simulink model "Test"  (R2021a)
settings: Solver=VariableStepAuto  StartTime=0.0  StopTime=10.0  RelTol=1e-3
values from neighbouring files (symbols this model uses):
  ff = 1.1    [Linearize_Fast.m]
  g = 9.81    [Linearize_Fast.m]    (also in Param_set.m = 9.8)
  ground_alt = 180.2070    (= 180.207)    [Linearize_Fast.m]
  m = 0.068    [Param_set.m]
  Mixer = double(subs(n_lin, [u_vec; a; b; c; d;], [.66708; 0; 0; 0;(1.86e-6);(8.856e-8);(8.856e-8);(9.766e-9)]))    [Linearize_Fast.m]
undefined symbols (not defined in the file or in its folder): all_cov, Discrete, K_PD, K_psi, K_u, K_v, Time
libraries: simulink x9, ctrlSharedLib x5
settings Model: Creator=jtc12  LastModifiedBy=jtc12

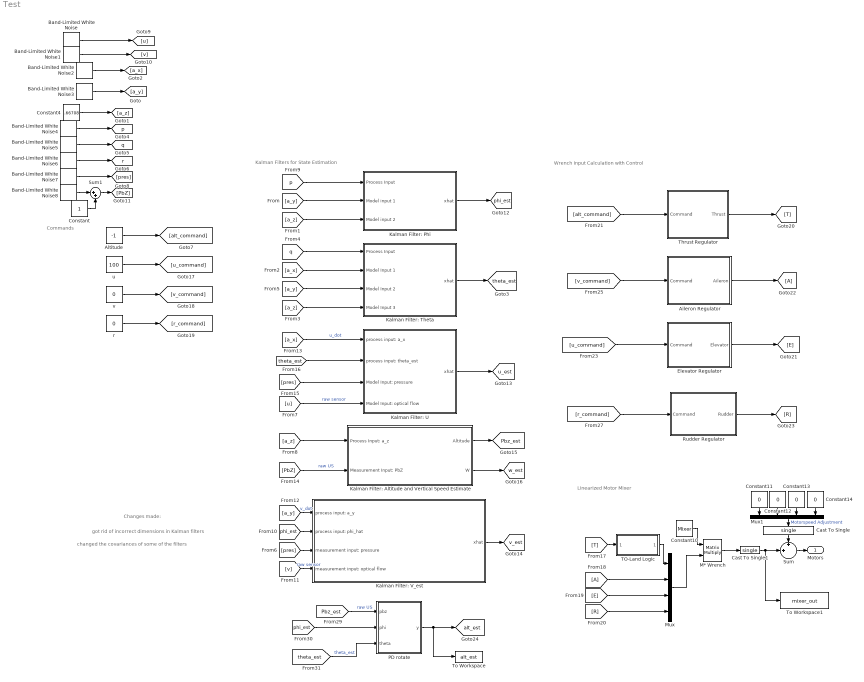
== system Test ==
  note: changed the covariances of some of the filters
  note: got rid of incorrect dimensions in Kalman filters
  note: Changes made:
  note: Commands
  note: Kalman Filters for State Estimation
  note: Wrench Input Calculation with Control
  note: Linearized Motor Mixer
  Aileron Regulator : Subsystem
  Altitude : Constant  Value=-1
  Band-Limited White Noise{,1..8} (9 alike) : simulink/Sources/Band-Limited White Noise  Cov=[0.1]  Ts=1/200  seed=[23341]
  Cast To Single : DataTypeConversion  OutDataTypeStr=single
  Cast To Single1 : DataTypeConversion  OutDataTypeStr=single
  Constant : Constant
  Constant10 : Constant  Value=Mixer
  Constant{11..14} (4 alike) : Constant  Value=0
  Constant4 : Constant  Value=.66708
  Elevator Regulator : Subsystem
  Kalman Filter: Altitude and Vertical Speed Estimate : Subsystem
  Kalman Filter: Phi : Subsystem
  Kalman Filter: Theta : Subsystem
  Kalman Filter: U : Subsystem
  Kalman Filter: V_est : Subsystem
  M* Wrench : Product  Multiplication=Matrix(*)
  Mux : Mux
  Mux1 : Mux
  PD rotate : MATLAB Function  TreatAsAtomicUnit=on
  Rudder Regulator : Subsystem
  Sum : Sum  Inputs=+|+||
  Sum1 : Sum  Inputs=|++
  TO-Land Logic : Subsystem
  Thrust Regulator : Subsystem
  To Workspace : ToWorkspace  VariableName=alt_est  SaveFormat=Timeseries  SampleTime=-1
  To Workspace1 : ToWorkspace  VariableName=mixer_out  SaveFormat=Timeseries  SampleTime=-1
  r : Constant  Value=0
  u : Constant  Value=100
  v : Constant  Value=0
  Motors : Outport  VectorParamsAs1DForOutWhenUnconnected=off
  tag scope: Pbz_est=global, alt_est=global, p=global, phi_est=global, q=global, r=global, theta_est=global, u_est=global, v_est=global, w_est=global
  wires:
  Band-Limited White Noise2/1 -> [a_x]
  Band-Limited White Noise3/1 -> [a_y]
  Constant4/1 -> [a_z]
  Band-Limited White Noise5/1 -> [q]
  Band-Limited White Noise6/1 -> [r]
  Band-Limited White Noise7/1 -> [pres]
  Altitude/1 -> [alt_command]
  v/1 -> [v_command]
  u/1 -> [u_command]
  r/1 -> [r_command]
  [phi_est] -> PD rotate/2(phi)
  [a_x] -> Kalman Filter: Theta/2(Model Input 1)
  Kalman Filter: Altitude and Vertical Speed Estimate/1(Altitude) -> [Pbz_est]
  Kalman Filter: V_est/1(xhat) -> [v_est]
  [PbZ] -> Kalman Filter: Altitude and Vertical Speed Estimate/2(Measurement Input: PbZ)  "raw US"
  [theta_est] -> PD rotate/3(theta)  "theta_est"
  Kalman Filter: Altitude and Vertical Speed Estimate/2(W) -> [w_est]
  [pres] -> Kalman Filter: V_est/3(measurement input: pressure)
  [Pbz_est] -> PD rotate/1(pbz)  "raw US"
  [a_y] -> Kalman Filter: Theta/3(Model Input 2)
  [a_z] -> Kalman Filter: Theta/4(Model Input 3)
  [a_y] -> Kalman Filter: Phi/2(Model input 1)
  [u] -> Kalman Filter: U/4(Model Input: optical flow)  "raw sensor"
  [pres] -> Kalman Filter: U/3(Model Input: pressure)
  [q] -> Kalman Filter: Theta/1(Process Input)
  Kalman Filter: U/1(xhat) -> [u_est]
  [a_y] -> Kalman Filter: V_est/1("process input: a_y   ")  "v_dot"
  [phi_est] -> Kalman Filter: V_est/2("process input: phi_hat ")
  [a_z] -> Kalman Filter: Altitude and Vertical Speed Estimate/1("Process Input: a_z ")
  Kalman Filter: Theta/1(xhat) -> [theta_est]
  [a_x] -> Kalman Filter: U/1(process input: a_x)  "u_dot"
  Kalman Filter: Phi/1(xhat) -> [phi_est]
  [theta_est] -> Kalman Filter: U/2(process input: theta_est)
  [a_z] -> Kalman Filter: Phi/3(Model input 2)
  PD rotate/1(y) -> To Workspace/1, [alt_est]
  [p] -> Kalman Filter: Phi/1(Process Input)
  [v] -> Kalman Filter: V_est/4(measurement input: optical flow)  "raw sensor"
  Rudder Regulator/1(Rudder) -> [R]
  Aileron Regulator/1(Aileron) -> [A]
  Thrust Regulator/1(Thrust) -> [T]
  [u_command] -> Elevator Regulator/1(Command)
  [alt_command] -> Thrust Regulator/1(Command)
  Elevator Regulator/1(Elevator) -> [E]
  [v_command] -> Aileron Regulator/1(Command)
  [r_command] -> Rudder Regulator/1(Command)
  Constant13/1 -> Mux1/3
  Constant12/1 -> Mux1/2
  Mux/1 -> M* Wrench/2
  [R] -> Mux/4
  Cast To Single1/1 -> Sum/2, To Workspace1/1
  Mux1/1 -> Cast To Single/1  "Motorspeed Adjustment"
  [E] -> Mux/3
  Cast To Single/1 -> Sum/1
  [T] -> TO-Land Logic/1(Thrust In)
  M* Wrench/1 -> Cast To Single1/1
  [A] -> Mux/2
  Constant10/1 -> M* Wrench/1
  Constant14/1 -> Mux1/4
  Sum/1 -> Motors/1
  TO-Land Logic/1(Thrust Out) -> Mux/1
  Constant11/1 -> Mux1/1
  Band-Limited White Noise/1 -> [u]
  Band-Limited White Noise1/1 -> [v]
  Band-Limited White Noise4/1 -> [p]
  Band-Limited White Noise8/1 -> Sum1/1
  Sum1/1 -> [PbZ]
  Constant/1 -> Sum1/2

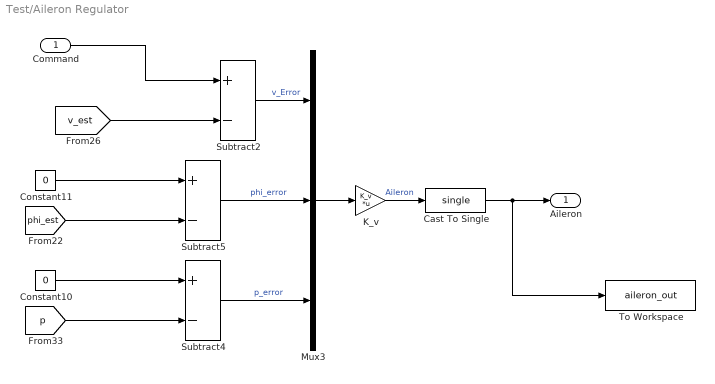
== system Test/Aileron Regulator ==
  Command : Inport
  Cast To Single : DataTypeConversion  OutDataTypeStr=single
  Constant10 : Constant  Value=0
  Constant11 : Constant  Value=0
  K_v : Gain  Gain=K_v  Multiplication=Matrix(K*u)
  Mux3 : Mux  Inputs=3
  Subtract2 : Sum  Inputs=+-
  Subtract4 : Sum  Inputs=+-
  Subtract5 : Sum  Inputs=+-
  To Workspace : ToWorkspace  VariableName=aileron_out  SaveFormat=Timeseries  SampleTime=-1
  Aileron : Outport
  wires:
  [p] -> Subtract4/2
  [v_est] -> Subtract2/2
  Constant11/1 -> Subtract5/1
  [phi_est] -> Subtract5/2
  Subtract5/1 -> Mux3/2  "phi_error"
  Subtract2/1 -> Mux3/1  "v_Error"
  Mux3/1 -> K_v/1
  Subtract4/1 -> Mux3/3  "p_error"
  Constant10/1 -> Subtract4/1
  K_v/1 -> Cast To Single/1  "Aileron"
  Command/1 -> Subtract2/1
  Cast To Single/1 -> To Workspace/1, Aileron/1

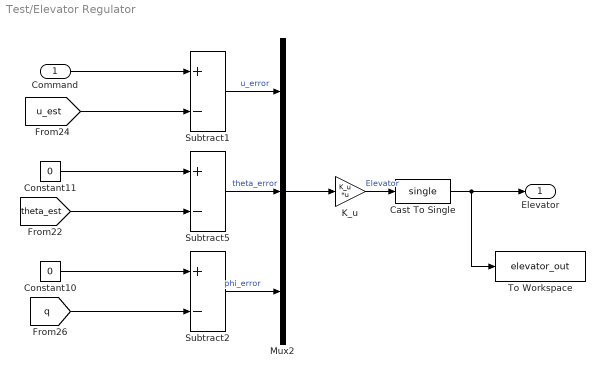
== system Test/Elevator Regulator ==
  Command : Inport
  Cast To Single : DataTypeConversion  OutDataTypeStr=single
  Constant10 : Constant  Value=0
  Constant11 : Constant  Value=0
  K_u : Gain  Gain=K_u  Multiplication=Matrix(K*u)
  Mux2 : Mux  Inputs=3
  Subtract1 : Sum  Inputs=+-
  Subtract2 : Sum  Inputs=+-
  Subtract5 : Sum  Inputs=+-
  To Workspace : ToWorkspace  VariableName=elevator_out  SaveFormat=Timeseries  SampleTime=-1
  Elevator : Outport
  wires:
  [theta_est] -> Subtract5/2
  [u_est] -> Subtract1/2
  Constant10/1 -> Subtract2/1
  Constant11/1 -> Subtract5/1
  Subtract5/1 -> Mux2/2  "theta_error"
  Subtract1/1 -> Mux2/1  "u_error"
  Subtract2/1 -> Mux2/3  "phi_error"
  Mux2/1 -> K_u/1
  [q] -> Subtract2/2
  K_u/1 -> Cast To Single/1  "Elevator"
  Command/1 -> Subtract1/1
  Cast To Single/1 -> To Workspace/1, Elevator/1

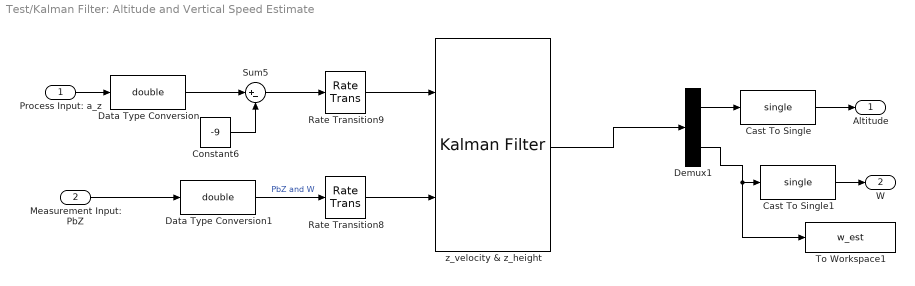
== system Test/Kalman Filter: Altitude and Vertical Speed Estimate ==
  "Process Input: a_z " : Inport
  Measurement Input: PbZ : Inport  Port=2
  Cast To Single : DataTypeConversion  OutDataTypeStr=single
  Cast To Single1 : DataTypeConversion  OutDataTypeStr=single
  Constant6 : Constant  Value=-9
  Data Type Conversion : DataTypeConversion  OutDataTypeStr=double
  Data Type Conversion1 : DataTypeConversion  OutDataTypeStr=double
  Demux1 : Demux  Outputs=2
  Rate Transition8 : RateTransition  OutPortSampleTime=1/200
  Rate Transition9 : RateTransition  OutPortSampleTime=1/200
  Sum5 : Sum  Inputs=|+-
  To Workspace1 : ToWorkspace  VariableName=w_est  SaveFormat=Timeseries  SampleTime=-1
  z_velocity & z_height : ctrlSharedLib/Kalman Filter  TimeDomain=Discrete-Time  UseCurrentEstimator=on  ModelSource=Individual A, B, C, D matrices  ModelSourceVariable=ss(0.95,1,1,0,1)  A=[1 1/200;0 1]  B=[0; 1/200]  C=[1 0]  D=0  NumberOfStates=1  NumberOfInputs=1  NumberOfOutputs=1  InitialEstimateSource=Dialog  X0=0  P0=10  UseK=off  UseGH=off  NumberOfProcessNoiseInputs=1  G=1  TimeInvariantG=on  H=0  TimeInvariantH=on  Q=all_cov(7,7)/1000  TimeInvariantQ=on  R=all_cov(1,1)  TimeInvariantR=on  N=0  TimeInvariantN=on  AddInputPort=on  AddEnablePort=off  OutputEstimatedY=off  OutputP=off  Ts=-1
  Altitude : Outport
  W : Outport  Port=2
  wires:
  Data Type Conversion1/1 -> Rate Transition8/1  "PbZ and W"
  Constant6/1 -> Sum5/2
  Demux1/1 -> Cast To Single/1
  Sum5/1 -> Rate Transition9/1
  Data Type Conversion/1 -> Sum5/1
  Rate Transition9/1 -> z_velocity & z_height/1
  Rate Transition8/1 -> z_velocity & z_height/2
  Measurement Input: PbZ/1 -> Data Type Conversion1/1
  Demux1/2 -> Cast To Single1/1, To Workspace1/1
  "Process Input: a_z "/1 -> Data Type Conversion/1
  z_velocity & z_height/1 -> Demux1/1
  Cast To Single/1 -> Altitude/1
  Cast To Single1/1 -> W/1

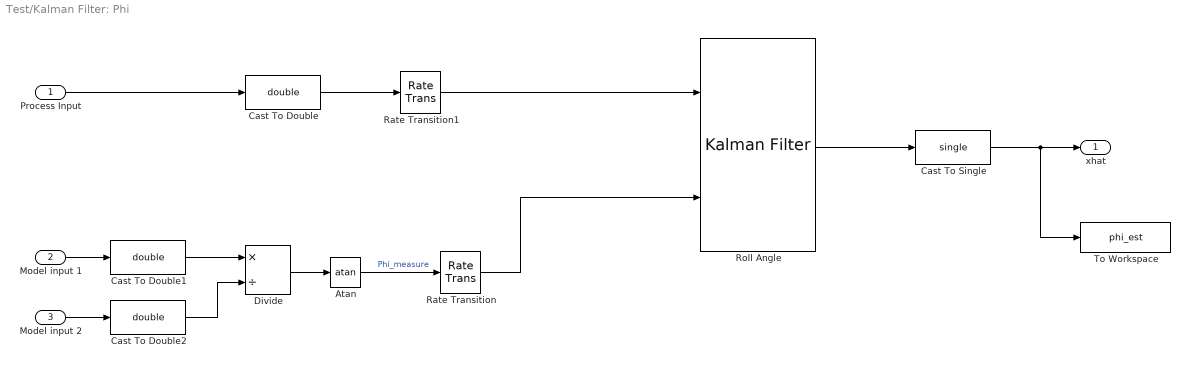
== system Test/Kalman Filter: Phi ==
  Process Input : Inport
  Model input 1 : Inport  Port=2
  Model input 2 : Inport  Port=3
  Atan : Trigonometry  Operator=atan
  Cast To Double : DataTypeConversion  OutDataTypeStr=double
  Cast To Double1 : DataTypeConversion  OutDataTypeStr=double
  Cast To Double2 : DataTypeConversion  OutDataTypeStr=double
  Cast To Single : DataTypeConversion  OutDataTypeStr=single
  Divide : Product  Inputs=*/
  Rate Transition : RateTransition  OutPortSampleTime=1/200
  Rate Transition1 : RateTransition  OutPortSampleTime=1/200
  Roll Angle : ctrlSharedLib/Kalman Filter  TimeDomain=Discrete-Time  UseCurrentEstimator=on  ModelSource=Individual A, B, C, D matrices  ModelSourceVariable=ss(0.95,1,1,0,1)  A=[1]  B=[1/200]  C=[1]  D=0  NumberOfStates=1  NumberOfInputs=1  NumberOfOutputs=1  InitialEstimateSource=Dialog  X0=0  P0=10  UseK=off  UseGH=off  NumberOfProcessNoiseInputs=1  G=1  TimeInvariantG=on  H=0  TimeInvariantH=on  Q=.0133/200  TimeInvariantQ=on  R=.0101  TimeInvariantR=on  N=0  TimeInvariantN=on  AddInputPort=on  AddEnablePort=off  OutputEstimatedY=off  OutputP=off  Ts=-1
  To Workspace : ToWorkspace  VariableName=phi_est  SaveFormat=Timeseries  SampleTime=-1
  xhat : Outport
  wires:
  Divide/1 -> Atan/1
  Atan/1 -> Rate Transition/1  "Phi_measure"
  Process Input/1 -> Cast To Double/1
  Rate Transition/1 -> Roll Angle/2
  Rate Transition1/1 -> Roll Angle/1
  Cast To Double/1 -> Rate Transition1/1
  Cast To Double1/1 -> Divide/1
  Model input 1/1 -> Cast To Double1/1
  Model input 2/1 -> Cast To Double2/1
  Cast To Double2/1 -> Divide/2
  Cast To Single/1 -> To Workspace/1, xhat/1
  Roll Angle/1 -> Cast To Single/1

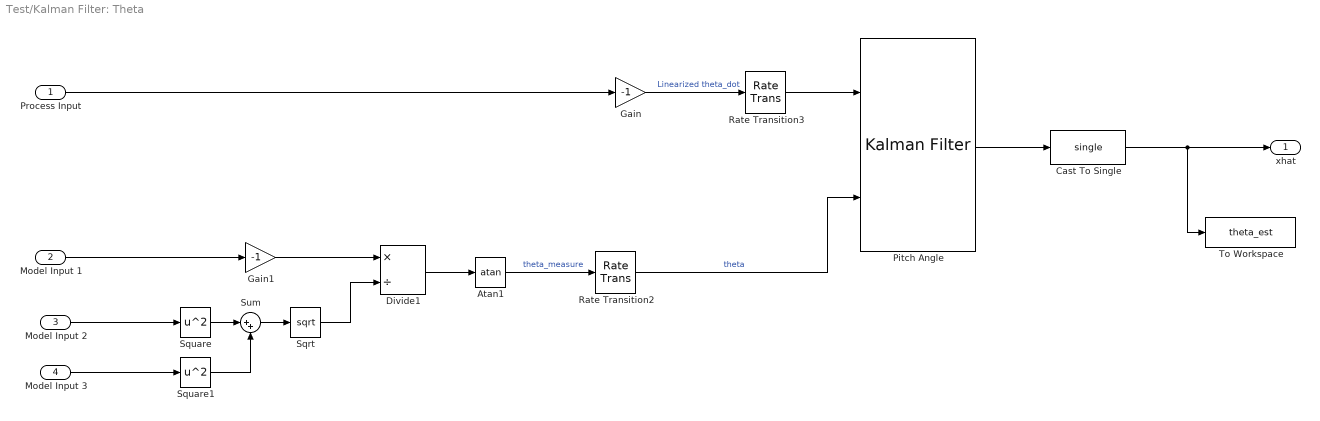
== system Test/Kalman Filter: Theta ==
  Process Input : Inport
  Model Input 1 : Inport  Port=2
  Model Input 2 : Inport  Port=3
  Model Input 3 : Inport  Port=4
  Atan1 : Trigonometry  Operator=atan
  Cast To Single : DataTypeConversion  OutDataTypeStr=single
  Divide1 : Product  Inputs=*/
  Gain : Gain  Gain=-1
  Gain1 : Gain  Gain=-1
  Pitch Angle : ctrlSharedLib/Kalman Filter  TimeDomain=Discrete-Time  UseCurrentEstimator=on  ModelSource=Individual A, B, C, D matrices  ModelSourceVariable=ss(0.95,1,1,0,1)  A=[1]  B=[1/200]  C=[1]  D=0  NumberOfStates=1  NumberOfInputs=1  NumberOfOutputs=1  InitialEstimateSource=Dialog  X0=0  P0=10  UseK=off  UseGH=off  NumberOfProcessNoiseInputs=1  G=1  TimeInvariantG=on  H=0  TimeInvariantH=on  Q=.0085/1000  TimeInvariantQ=on  R=.0066/10  TimeInvariantR=on  N=0  TimeInvariantN=on  AddInputPort=on  AddEnablePort=off  OutputEstimatedY=off  OutputP=off  Ts=-1
  Rate Transition2 : RateTransition  OutPortSampleTime=1/200
  Rate Transition3 : RateTransition  OutPortSampleTime=1/200
  Sqrt : Sqrt  SaturateOnIntegerOverflow=on
  Square : Math  Operator=square  SaturateOnIntegerOverflow=on
  Square1 : Math  Operator=square  SaturateOnIntegerOverflow=on
  Sum : Sum  Inputs=|++
  To Workspace : ToWorkspace  VariableName=theta_est  SaveFormat=Timeseries  SampleTime=-1
  xhat : Outport
  wires:
  Gain1/1 -> Divide1/1
  Divide1/1 -> Atan1/1
  Model Input 2/1 -> Square/1
  Rate Transition3/1 -> Pitch Angle/1
  Sum/1 -> Sqrt/1
  Square/1 -> Sum/1
  Square1/1 -> Sum/2
  Atan1/1 -> Rate Transition2/1  "theta_measure"
  Sqrt/1 -> Divide1/2
  Rate Transition2/1 -> Pitch Angle/2  "theta"
  Gain/1 -> Rate Transition3/1  "Linearized theta_dot"
  Process Input/1 -> Gain/1
  Model Input 1/1 -> Gain1/1
  Model Input 3/1 -> Square1/1
  Cast To Single/1 -> xhat/1, To Workspace/1
  Pitch Angle/1 -> Cast To Single/1

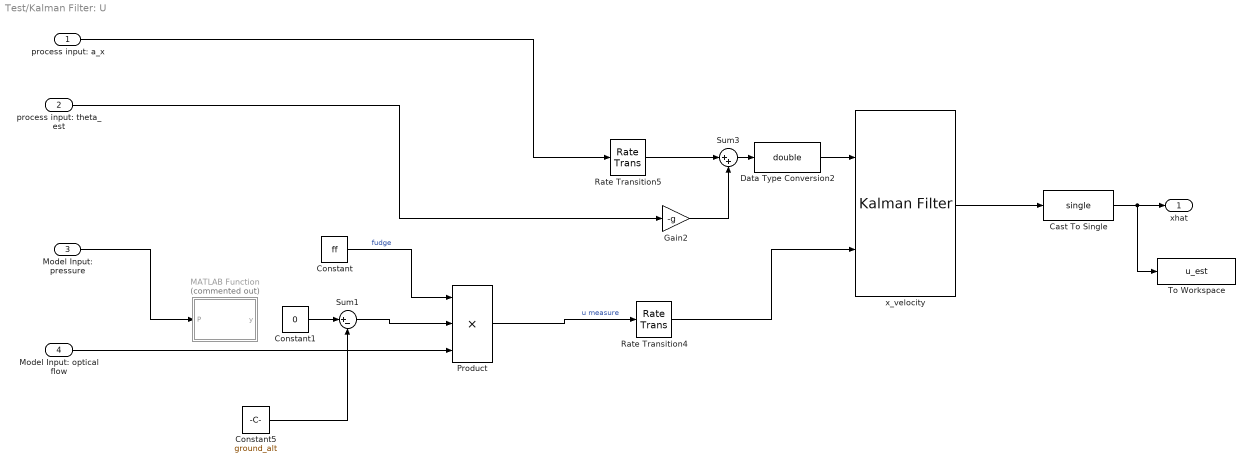
== system Test/Kalman Filter: U ==
  process input: a_x : Inport
  process input: theta_est : Inport  Port=2
  Model Input: pressure : Inport  Port=3
  Model Input: optical flow : Inport  Port=4
  Cast To Single : DataTypeConversion  OutDataTypeStr=single
  Constant : Constant  Value=ff
  Constant1 : Constant  Value=0
  Constant5 : Constant  Value=ground_alt
  Data Type Conversion2 : DataTypeConversion  OutDataTypeStr=double
  Gain2 : Gain  Gain=-g
  MATLAB Function : MATLAB Function  Commented=on  TreatAsAtomicUnit=on
  Product : Product  Inputs=3
  Rate Transition4 : RateTransition  OutPortSampleTime=1/200
  Rate Transition5 : RateTransition  OutPortSampleTime=1/200
  Sum1 : Sum  Inputs=|+-
  Sum3 : Sum  Inputs=|++
  To Workspace : ToWorkspace  VariableName=u_est  SaveFormat=Timeseries  SampleTime=-1
  x_velocity : ctrlSharedLib/Kalman Filter  TimeDomain=Discrete-Time  UseCurrentEstimator=on  ModelSource=Individual A, B, C, D matrices  ModelSourceVariable=ss(0.95,1,1,0,1)  A=[1]  B=[1/200]  C=[1]  D=0  NumberOfStates=1  NumberOfInputs=1  NumberOfOutputs=1  InitialEstimateSource=Dialog  X0=0  P0=10  UseK=off  UseGH=off  NumberOfProcessNoiseInputs=1  G=1  TimeInvariantG=on  H=0  TimeInvariantH=on  Q=.0059/200  TimeInvariantQ=on  R=all_cov(10,8)  TimeInvariantR=on  N=0  TimeInvariantN=on  AddInputPort=on  AddEnablePort=off  OutputEstimatedY=off  OutputP=off  Ts=-1
  xhat : Outport
  wires:
  process input: theta_est/1 -> Gain2/1
  Gain2/1 -> Sum3/2
  Product/1 -> Rate Transition4/1  "u measure"
  Rate Transition4/1 -> x_velocity/2
  process input: a_x/1 -> Rate Transition5/1
  Rate Transition5/1 -> Sum3/1
  Sum1/1 -> Product/2
  Data Type Conversion2/1 -> x_velocity/1
  Constant/1 -> Product/1  "fudge"
  Sum3/1 -> Data Type Conversion2/1
  Constant5/1 -> Sum1/2
  Model Input: pressure/1 -> MATLAB Function/1(P)
  Model Input: optical flow/1 -> Product/3
  Cast To Single/1 -> To Workspace/1, xhat/1
  x_velocity/1 -> Cast To Single/1
  Constant1/1 -> Sum1/1

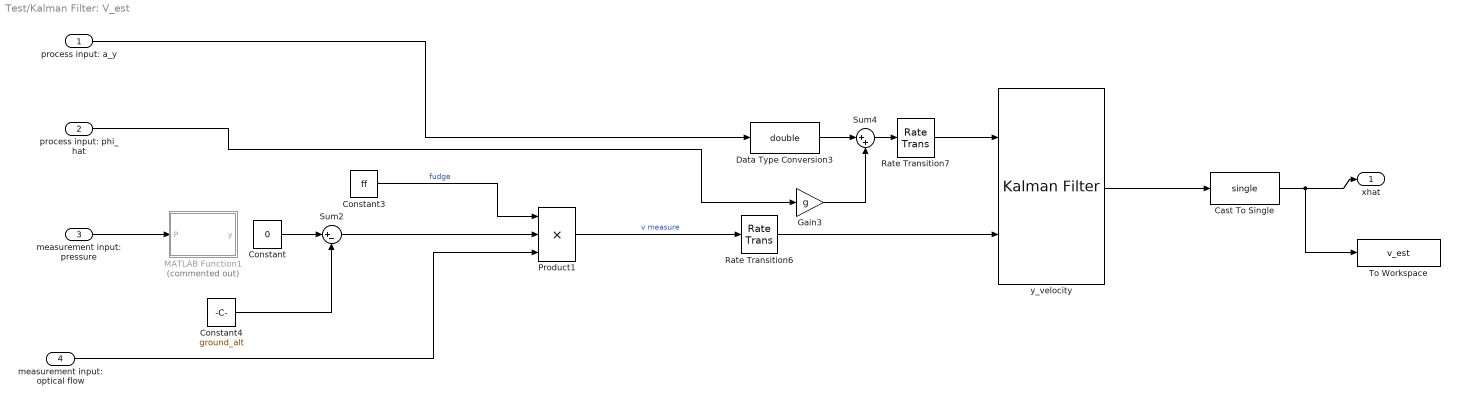
== system Test/Kalman Filter: V_est ==
  "process input: a_y   " : Inport
  "process input: phi_hat " : Inport  Port=2
  measurement input: pressure : Inport  Port=3
  measurement input: optical flow : Inport  Port=4
  Cast To Single : DataTypeConversion  OutDataTypeStr=single
  Constant : Constant  Value=0
  Constant3 : Constant  Value=ff
  Constant4 : Constant  Value=ground_alt
  Data Type Conversion3 : DataTypeConversion  OutDataTypeStr=double
  Gain3 : Gain  Gain=g
  MATLAB Function1 : MATLAB Function  Commented=on  TreatAsAtomicUnit=on
  Product1 : Product  Inputs=3
  Rate Transition6 : RateTransition  OutPortSampleTime=1/200
  Rate Transition7 : RateTransition  OutPortSampleTime=1/200
  Sum2 : Sum  Inputs=|+-
  Sum4 : Sum  Inputs=|++
  To Workspace : ToWorkspace  VariableName=v_est  SaveFormat=Timeseries  SampleTime=-1
  y_velocity : ctrlSharedLib/Kalman Filter  TimeDomain=Discrete-Time  UseCurrentEstimator=on  ModelSource=Individual A, B, C, D matrices  ModelSourceVariable=ss(0.95,1,1,0,1)  A=[1]  B=[1/200]  C=[1]  D=0  NumberOfStates=1  NumberOfInputs=1  NumberOfOutputs=1  InitialEstimateSource=Dialog  X0=0  P0=10  UseK=off  UseGH=off  NumberOfProcessNoiseInputs=1  G=1  TimeInvariantG=on  H=0  TimeInvariantH=on  Q=.0087/200  TimeInvariantQ=on  R=2.5  TimeInvariantR=on  N=0  TimeInvariantN=on  AddInputPort=on  AddEnablePort=off  OutputEstimatedY=off  OutputP=off  Ts=-1
  xhat : Outport
  wires:
  Gain3/1 -> Sum4/2
  Sum2/1 -> Product1/2
  measurement input: optical flow/1 -> Product1/3
  Constant4/1 -> Sum2/2
  Product1/1 -> Rate Transition6/1  "v measure"
  Rate Transition6/1 -> y_velocity/2
  Sum4/1 -> Rate Transition7/1
  Constant3/1 -> Product1/1  "fudge"
  Rate Transition7/1 -> y_velocity/1
  Data Type Conversion3/1 -> Sum4/1
  "process input: phi_hat "/1 -> Gain3/1
  measurement input: pressure/1 -> MATLAB Function1/1(P)
  "process input: a_y   "/1 -> Data Type Conversion3/1
  y_velocity/1 -> Cast To Single/1
  Cast To Single/1 -> xhat/1, To Workspace/1
  Constant/1 -> Sum2/1

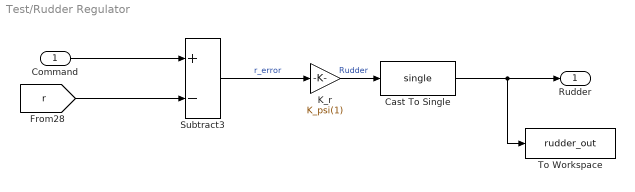
== system Test/Rudder Regulator ==
  Command : Inport
  Cast To Single : DataTypeConversion  OutDataTypeStr=single
  K_r : Gain  Gain=K_psi(1)
  Subtract3 : Sum  Inputs=+-
  To Workspace : ToWorkspace  VariableName=rudder_out  SaveFormat=Timeseries  SampleTime=-1
  Rudder : Outport
  wires:
  Subtract3/1 -> K_r/1  "r_error"
  K_r/1 -> Cast To Single/1  "Rudder"
  [r] -> Subtract3/2
  Command/1 -> Subtract3/1
  Cast To Single/1 -> To Workspace/1, Rudder/1

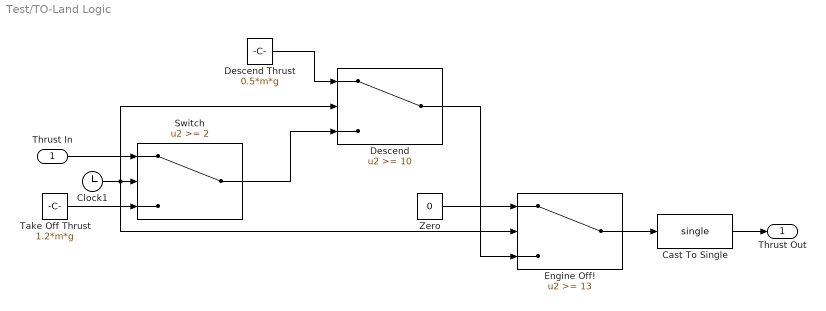
== system Test/TO-Land Logic ==
  Thrust In : Inport
  Cast To Single : DataTypeConversion  OutDataTypeStr=single
  Clock1 : Clock
  Descend : Switch  Threshold=10
  Descend Thrust : Constant  Value=0.5*m*g
  Engine Off! : Switch  Threshold=13
  Switch : Switch  Threshold=2
  Take Off Thrust : Constant  Value=1.2*m*g
  Zero : Constant  Value=0
  Thrust Out : Outport
  wires:
  Take Off Thrust/1 -> Switch/3
  Clock1/1 -> Engine Off!/2, Descend/2, Switch/2
  Thrust In/1 -> Switch/1
  Switch/1 -> Descend/3
  Descend Thrust/1 -> Descend/1
  Descend/1 -> Engine Off!/3
  Zero/1 -> Engine Off!/1
  Engine Off!/1 -> Cast To Single/1
  Cast To Single/1 -> Thrust Out/1

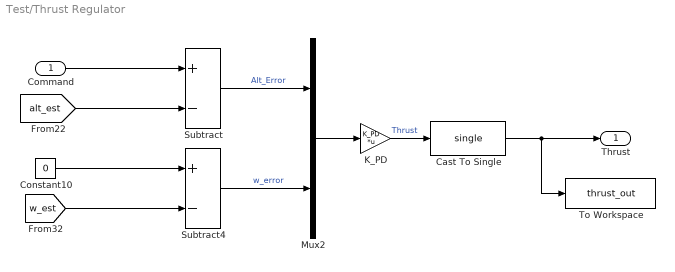
== system Test/Thrust Regulator ==
  Command : Inport
  Cast To Single : DataTypeConversion  OutDataTypeStr=single
  Constant10 : Constant  Value=0
  K_PD : Gain  Gain=K_PD  Multiplication=Matrix(K*u)
  Mux2 : Mux  Inputs=2
  Subtract : Sum  Inputs=+-
  Subtract4 : Sum  Inputs=+-
  To Workspace : ToWorkspace  VariableName=thrust_out  SaveFormat=Timeseries  SampleTime=-1
  Thrust : Outport
  wires:
  Subtract4/1 -> Mux2/2  "w_error"
  [w_est] -> Subtract4/2
  [alt_est] -> Subtract/2
  Subtract/1 -> Mux2/1  "Alt_Error"
  K_PD/1 -> Cast To Single/1  "Thrust"
  Command/1 -> Subtract/1
  Constant10/1 -> Subtract4/1
  Mux2/1 -> K_PD/1
  Cast To Single/1 -> To Workspace/1, Thrust/1

== matlab function Test/Kalman Filter: U/MATLAB Function ==
  data: P input; y output
function y = z_pres(P)
g = 9.8; % acceleration due to gravity m/s^2
M = 0.0289644; % molar mass of air in kg/mol
R = 8.31432; % universal gas constant Nm/mol/k
p0 = 101325; % Pa standard pressure

T =288.15;  % Assumed temperature in kelvin
K =-g*M/R/T;
z_hypsometric = 1/K*log(P/p0);
y = z_hypsometric;

== matlab function Test/PD rotate ==
  data: pbz input; y output; phi input; theta input
function y = rotate_BE(pbz, phi, theta)
roll_BE = [1 0 0; 0 cos(phi) sin(phi); 0 -sin(phi) cos(phi)]';
pitch_BE = [cos(theta) 0 -sin(theta); 0 1 0; sin(theta) 0 cos(theta);]';
%yaw_BE = simplify(inv([cos(psi) sin(psi) 0; -sin(psi) cos(psi) 0; 0 0 1;]));
rotater = roll_BE*pitch_BE*pbz;
y = rotater(3);

== matlab function Test/Kalman Filter: V_est/MATLAB Function1 ==
  data: P input; y output
function y = z_pres(P)
g = 9.8; % acceleration due to gravity m/s^2
M = 0.0289644; % molar mass of air in kg/mol
R = 8.31432; % universal gas constant Nm/mol/k
p0 = 101325; % Pa standard pressure

T =288.15;  % Assumed temperature in kelvin
K =-g*M/R/T;
z_hypsometric = 1/K*log(P/p0);
y = z_hypsometric;
